simulink model "UDP"  (R2019a)
settings: Solver=VariableStepAuto  StartTime=0.0  StopTime=inf  RelTol=1e-3
undefined symbols (not defined in the file): f
libraries: aerolibconvert2 x3, xpcutilitieslib x2, instrumentlib x2
settings Model: Creator=10291  LastModifiedBy=10291

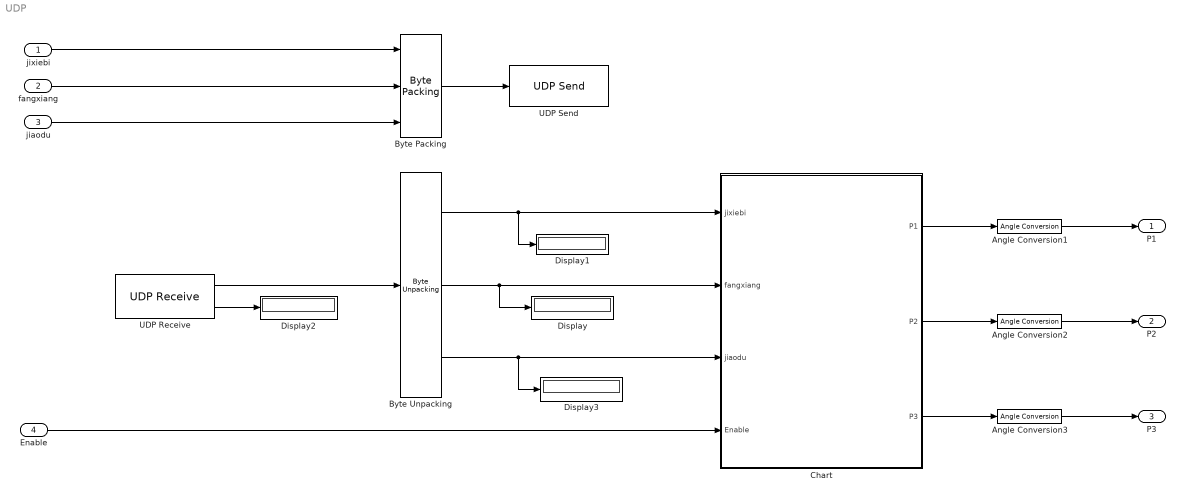
== system UDP ==
  jixiebi : Inport
  fangxiang : Inport  Port=2
  jiaodu : Inport  Port=3
  Enable : Inport  Port=4
  Angle Conversion1 : aerolibconvert2/Angle Conversion  IU=deg  OU=rad
  Angle Conversion2 : aerolibconvert2/Angle Conversion  IU=deg  OU=rad
  Angle Conversion3 : aerolibconvert2/Angle Conversion  IU=deg  OU=rad
  "Byte Packing " : xpcutilitieslib/Byte Packing   MaskPackedDataType=double  MaskUnpackedDataTypes={'uint8','uint8','uint8'}  MaskAlignment=1
  "Byte Unpacking " : xpcutilitieslib/Byte Unpacking   MaskUnpackedDataTypes={'uint8','uint8','uint8'}  MaskUnpackedDataSizes={[1],[1],[1]}  MaskAlignment=1
      settings: SourceProductName=Simulink Real-Time  SourceProductBaseCode=XP
  Chart : Stateflow chart  TreatAsAtomicUnit=on
  Display{,1..3} (4 alike) : Display
  UDP Receive : instrumentlib/UDP Receive  Priority=3  Host=localhost  Port=51000  LocalPort=51001  EnablePortSharing=off  GetLatestData=off  DataSize=[1 1]  DataType=double  ASCIIFormatting=%f,  Terminator=LF  ByteOrder=BigEndian  EnableBlockingMode=off  Timeout=5  SampleTime=0.1  LocalAddress=0.0.0.0
      settings: SourceProductName=Instrument Control Toolbox
  UDP Send : instrumentlib/UDP Send  Priority=2  Host=localhost  Port=51001  LocalPort=51000  EnablePortSharing=off  ByteOrder=BigEndian  OutputDatagramPacketSize=10  EnableBlockingMode=on  LocalAddress=0.0.0.0
      settings: SourceProductName=Instrument Control Toolbox
  P1 : Outport
  P2 : Outport  Port=2
  P3 : Outport  Port=3
  wires:
  "Byte Packing "/1 -> UDP Send/1
  "Byte Unpacking "/1 -> Chart/1(jixiebi), Display1/1
  "Byte Unpacking "/2 -> Display/1, Chart/2(fangxiang)
  UDP Receive/1 -> "Byte Unpacking "/1
  UDP Receive/2 -> Display2/1
  "Byte Unpacking "/3 -> Display3/1, Chart/3(jiaodu)
  Chart/3(P3) -> Angle Conversion3/1
  Chart/2(P2) -> Angle Conversion2/1
  Chart/1(P1) -> Angle Conversion1/1
  Angle Conversion2/1 -> P2/1
  Angle Conversion3/1 -> P3/1
  Angle Conversion1/1 -> P1/1
  Enable/1 -> Chart/4(Enable)
  jixiebi/1 -> "Byte Packing "/1
  fangxiang/1 -> "Byte Packing "/2
  jiaodu/1 -> "Byte Packing "/3

== stateflow chart UDP/Chart ==
  (default) -> (junction 60)
  (junction 60) -> (junction 3) [order 1] : [hasChangedTo(Enable,1)]
  (junction 3) -> (junction 9) [order 1] : [jixiebi  == 1]
  (junction 9) -> (junction 18) [order 1] : [fangxiang == 1]
  (junction 60) -> (junction 62) [order 2]
  (junction 3) -> (junction 23) [order 2]
  (junction 9) -> (junction 12) [order 2] : {
      | P1 = P1 - jiaodu;
      | }
  (junction 18) -> (junction 20) : {
      | P1 = P1 + jiaodu;
      | }
  (junction 12) -> (junction 23)
  (junction 20) -> (junction 12)
  (junction 23) -> (junction 29)
  (junction 29) -> (junction 32) [order 1] : [jixiebi  == 2]
  (junction 32) -> (junction 35) [order 1] : [fangxiang == 1]
  (junction 29) -> (junction 26) [order 2]
  (junction 32) -> (junction 31) [order 2] : {
      | P2 = P2 - jiaodu;
      | }
  (junction 35) -> (junction 38) : {
      | P2 = P2 + jiaodu;
      | }
  (junction 31) -> (junction 26)
  (junction 38) -> (junction 31)
  (junction 26) -> (junction 43)
  (junction 43) -> (junction 46) [order 1] : [jixiebi  == 3]
  (junction 46) -> (junction 49) [order 1] : [fangxiang == 1]
  (junction 43) -> (junction 40) [order 2]
  (junction 46) -> (junction 45) [order 2] : {
      | P3 = P3 - jiaodu;
      | }
  (junction 49) -> (junction 52) : {
      | P3 = P3 + jiaodu;
      | }
  (junction 40) -> (junction 62)
  (junction 45) -> (junction 40)
  (junction 52) -> (junction 45)
  (junction 62) -> (junction 54)
  (junction 54) -> (junction 65) [order 1] : [jixiebi == 0]
  (junction 54) -> (junction 69) [order 2]
  (junction 65) -> (junction 67) : {
      | P1 = 0;
      | P2 = 0;
      | P3 = 0;
      | }
  (junction 67) -> (junction 69)
  (junction 69) -> (junction 72)
  data: jixiebi input size=1; P1 output; P2 output double; P3 output double; fangxiang input; jiaodu input; Enable input
